simulink model "PV_MEV_FFT_HGQ_BLS"  (R2025a)
settings: Solver=VariableStepAuto  StartTime=0.0  StopTime=0.15  RelTol=1e-3
InitFcn:
  | init_paras
model workspace (MAT data in the model file):
  atk_params = [0 1 0.08 999 0 50 0 0]
values from neighbouring files (symbols this model uses):
  C_PFC = 2600e-6    (= 0.0026)    [init_paras.m]
  ENABLE_HIL = 0    [init_paras.m]
  estimation_src = 1    [init_paras.m]
  Fnom = 50    [init_paras.m]
  Fr_I = Fnom*2    (= 100)    [init_paras.m]
  Ki_V = 80    [init_paras.m]
  Kp_I = 0.06    [init_paras.m]
  Kp_V = 0.25    [init_paras.m]
  Kr_I = 2.5    [init_paras.m]
  L_PFC = 600e-6    (= 0.0006)    [init_paras.m]
  Limit_V = 100    [init_paras.m]
  mm_10cycle_points = mm_points_per_cycle * 10    (= 800)    [init_paras.m]
  mm_fund_freq = 50    [init_paras.m]
  mm_points_per_cycle = 80    [init_paras.m]
  RL_PFC = 20e-3    (= 0.02)    [init_paras.m]
  Ro = 22.22    [init_paras.m]
  Ts_Control = 1/Fc    (= 1e-05)    [init_paras.m]
  Ts_Power = 50e-9    (= 5e-08)    [init_paras.m]
  use_d_predict = 1    [init_paras.m]
  use_harmonic = 1    [init_paras.m]
  use_p_predict = 0    [init_paras.m]
  Vnom_ac = 240    [init_paras.m]
undefined symbols (not defined in the file or in its folder): D1, Delta, DiscIntNeverNeededParam
libraries: spsSeriesRLCBranchLib x17, spsMeanLib x16, spsCurrentMeasurementLib x9, spsFourierLib x8, spsTHDLib x8, spsVoltageMeasurementLib x8, spsDiodeLib x7, MyLibrary x6, instrumentlib x6, pycoexlib x6, simulink x6, spsPWMGeneratorDCDCLib x4
(part 6 of 6)

== matlab function PV_MEV_FFT_HGQ_BLS/EV System2/PFC Control/D_predict ==
  data: i_L input; D output; i_ref input; V_in input; Ts input; L_in input; V_o input; theta_pll input; amp_est input; phase_est input; use_harmonic input
function D  = fcn(i_L, i_ref, V_in, Ts, L_in, V_o, theta_pll, amp_est, phase_est, use_harmonic)

    persistent theta_prev;
    if isempty(theta_prev)
        theta_prev = theta_pll;
    end

    % hyper parameters
    track_gain = 0.35;
    damp_gain = 0.015;

    % Optional
    lead_steps = 1.0;


    % Initialisation 
    L = max(L_in, 1e-9);
    Ts_eff = max(Ts, 1e-9);
    Vo = max(abs(V_o), 1.0);
    ui_L = abs(i_L);

    if V_in > 0
        line_sign = 1.0;
    else
        line_sign = -1.0;
    end

    i_ref_signed = line_sign * abs(i_ref);

    plant_gain = line_sign * L / (Vo * Ts_eff);
    D_ff = 1.0 - abs(V_in) / Vo;

    if use_harmonic

        dtheta = atan2(sin(theta_pll - theta_prev), cos(theta_pll - theta_prev));
        theta_prev = theta_pll;

        omega_inst = dtheta / Ts_eff;

        theta_ctrl = theta_pll + omega_inst * Ts_eff * lead_steps;

        A3 = abs(amp_est(2));
        A5 = abs(amp_est(3));
        A7 = abs(amp_est(4));

        phi3 = phase_est(1);
        phi5 = phase_est(2);
        phi7 = phase_est(3);

        phase_sign = 1.0;

        ih3 = A3 * sin(3.0 * theta_ctrl + phase_sign * phi3);
        ih5 = A5 * sin(5.0 * theta_ctrl + phase_sign * phi5);
        ih7 = A7 * sin(7.0 * theta_ctrl + phase_sign * phi7);

        k3 = 1.00;
        k5 = 1.08;
        k7 = 1.00;

        ih_357 = k3 * ih3 + k5 * ih5 + k7 * ih7;

        i_ref_signed = i_ref_signed - ih_357;
    end

    i_err = i_ref_signed - i_L;

    D_corr = plant_gain * track_gain * i_err;
    D_damp = -line_sign * damp_gain * (i_L - i_ref_signed) / ui_L;

    D = D_ff + D_corr + D_damp;
end

== matlab function PV_MEV_FFT_HGQ_BLS/EV System2/PFC Control/Half Cycle Model Prediction/MATLAB Function ==
  data: x input; x_norm output; A output
function [x_norm, A] = CycleNorm(x)
A = max(abs(x));
A = max(A, 1e-6);
x_norm = x / A;

== matlab function PV_MEV_FFT_HGQ_BLS/EV System/PFC Control/D_predict ==
  data: i_L input; D output; i_ref input; V_in input; Ts input; L_in input; V_o input; theta_pll input; amp_est input; phase_est input; use_harmonic input
function D  = fcn(i_L, i_ref, V_in, Ts, L_in, V_o, theta_pll, amp_est, phase_est, use_harmonic)

    persistent theta_prev;
    if isempty(theta_prev)
        theta_prev = theta_pll;
    end

    % hyper parameters
    track_gain = 0.35;
    damp_gain = 0.015;

    % Optional
    lead_steps = 1.0;


    % Initialisation 
    L = max(L_in, 1e-9);
    Ts_eff = max(Ts, 1e-9);
    Vo = max(abs(V_o), 1.0);
    ui_L = max(abs(i_L), 1e-6);

    if V_in > 0
        line_sign = 1.0;
    else
        line_sign = -1.0;
    end

    i_ref_signed = line_sign * abs(i_ref);

    plant_gain = line_sign * L / (Vo * Ts_eff);
    D_ff = 1.0 - abs(V_in) / Vo;

    if use_harmonic

        dtheta = atan2(sin(theta_pll - theta_prev), cos(theta_pll - theta_prev));
        theta_prev = theta_pll;

        omega_inst = dtheta / Ts_eff;

        theta_ctrl = theta_pll + omega_inst * Ts_eff * lead_steps;

        A3 = abs(amp_est(2));
        A5 = abs(amp_est(3));
        A7 = abs(amp_est(4));

        phi3 = phase_est(1);
        phi5 = phase_est(2);
        phi7 = phase_est(3);

        phase_sign = 1.0;

        ih3 = A3 * sin(3.0 * theta_ctrl + phase_sign * phi3);
        ih5 = A5 * sin(5.0 * theta_ctrl + phase_sign * phi5);
        ih7 = A7 * sin(7.0 * theta_ctrl + phase_sign * phi7);

        k3 = 1.00;
        k5 = 1.08;
        k7 = 1.00;

        ih_357 = k3 * ih3 + k5 * ih5 + k7 * ih7;

        i_ref_signed = i_ref_signed - ih_357;
    end

    i_err = i_ref_signed - i_L;

    D_corr = plant_gain * track_gain * i_err;
    D_damp = -line_sign * damp_gain * (i_L - i_ref_signed) / ui_L;

    D = D_ff + D_corr + D_damp;
end

== matlab function PV_MEV_FFT_HGQ_BLS/EV System/PFC Control/fft estimation 1 cycle2/FFT_estimation_1 ==
  data: u input; amp output; phase output; fs input; f0 input
function [amp, phase] = FFT_estimation_1(u, fs, f0)
%#codegen

x = double(u(:));
N = length(x);

h = zeros(4, 1);
h(1) = 1;
h(2) = 3;
h(3) = 5;
h(4) = 7;

X = fft(x);

amp = zeros(4, 1);
phase_abs_sin = zeros(4, 1);
phase = zeros(3, 1);

tol = 1e-12;

for i = 1:4
    harmonicOrder = h(i);

    bin = round(harmonicOrder * f0 * double(N) / fs);

    if bin <= 0 || bin > floor(double(N) / 2)
        amp(i) = 0;
        phase_abs_sin(i) = 0;
    else
        idx = int32(bin + 1);
        C = X(idx);

        if mod(N, 2) == 0 && bin == N / 2
            amp(i) = abs(C) / double(N);
        else
            amp(i) = 2 * abs(C) / double(N);
        end

        if amp(i) < tol
            phase_abs_sin(i) = 0;
        else
            ph_raw = angle(C);

            ph_sin = ph_raw + pi/2;

            phase_abs_sin(i) = atan2(sin(ph_sin), cos(ph_sin));
        end
    end
end

if amp(1) < tol
    phase(1) = 0;
    phase(2) = 0;
    phase(3) = 0;
else
    phase(1) = atan2( ...
        sin(phase_abs_sin(2) - 3 * phase_abs_sin(1)), ...
        cos(phase_abs_sin(2) - 3 * phase_abs_sin(1)) ...
    );

    phase(2) = atan2( ...
        sin(phase_abs_sin(3) - 5 * phase_abs_sin(1)), ...
        cos(phase_abs_sin(3) - 5 * phase_abs_sin(1)) ...
    );

    phase(3) = atan2( ...
        sin(phase_abs_sin(4) - 7 * phase_abs_sin(1)), ...
        cos(phase_abs_sin(4) - 7 * phase_abs_sin(1)) ...
    );
end

end

== matlab function PV_MEV_FFT_HGQ_BLS/EV System/PFC Control/fft estimation 10 cycle2/FFT_estimation ==
  data: u input; amp output; phase output; fs input; f0 input
function [amp, phase] = FFT_estimation(u, fs, f0)
%#codegen

x = double(u(:));
N = length(x);

h = zeros(4, 1);
h(1) = 1;
h(2) = 3;
h(3) = 5;
h(4) = 7;

X = fft(x);

amp = zeros(4, 1);
phase_abs_sin = zeros(4, 1);
phase = zeros(3, 1);

tol = 1e-12;

for i = 1:4
    harmonicOrder = h(i);

    bin = round(harmonicOrder * f0 * double(N) / fs);

    if bin <= 0 || bin > floor(double(N) / 2)
        amp(i) = 0;
        phase_abs_sin(i) = 0;
    else
        idx = int32(bin + 1);
        C = X(idx);

        if mod(N, 2) == 0 && bin == N / 2
            amp(i) = abs(C) / double(N);
        else
            amp(i) = 2 * abs(C) / double(N);
        end

        if amp(i) < tol
            phase_abs_sin(i) = 0;
        else
            ph_raw = angle(C);

            ph_sin = ph_raw + pi/2;

            phase_abs_sin(i) = atan2(sin(ph_sin), cos(ph_sin));
        end
    end
end

if amp(1) < tol
    phase(1) = 0;
    phase(2) = 0;
    phase(3) = 0;
else
    phase(1) = atan2( ...
        sin(phase_abs_sin(2) - 3 * phase_abs_sin(1)), ...
        cos(phase_abs_sin(2) - 3 * phase_abs_sin(1)) ...
    );

    phase(2) = atan2( ...
        sin(phase_abs_sin(3) - 5 * phase_abs_sin(1)), ...
        cos(phase_abs_sin(3) - 5 * phase_abs_sin(1)) ...
    );

    phase(3) = atan2( ...
        sin(phase_abs_sin(4) - 7 * phase_abs_sin(1)), ...
        cos(phase_abs_sin(4) - 7 * phase_abs_sin(1)) ...
    );
end

end

== matlab function PV_MEV_FFT_HGQ_BLS/EV System/PFC Control/One  Cycle Model Prediction/MATLAB Function ==
  data: x input; x_norm output; A output
function [x_norm, A] = CycleNorm(x)
A = max(abs(x));
A = max(A, 1e-6);
x_norm = x / A;

== matlab function PV_MEV_FFT_HGQ_BLS/EV System2/PFC Control/Half Cycle Model Prediction/MATLAB Function3 ==
  data: y_rel input; y_post output; A_latest input; alpha input; reset input
function y_post = harmonic_postprocess(y_rel, A_latest, alpha, reset)
%#codegen
% 一体化后处理：
% 1) EMA 平滑（在相对输出域）
% 2) A 恢复（幅值乘 A）
% 3) atan2 恢复相位（由 cos/sin -> phase）
%
% 输入:
%   y_rel    : 模型输出(10x1 或 1x10)
%              [amp_h1_rel, amp_h3_rel, amp_h5_rel, amp_h7_rel, ...
%               cos_h3, sin_h3, cos_h5, sin_h5, cos_h7, sin_h7]
%   A_latest : A 恢复系数（可标量或向量；向量时自动取 max(abs(.))）
%   alpha    : EMA 系数 [0,1]，建议 0.10~0.16
%   reset    : 复位信号（true 时重置 EMA 状态）
%
% 输出:
%   y_post(7x1):
%   [amp_h1_abs, amp_h3_abs, amp_h5_abs, amp_h7_abs, phase_h3, phase_h5, phase_h7]

persistent ema_state initialized
if isempty(initialized)
    ema_state = zeros(10,1,'single');
    initialized = false;
end

% -------- 参数/输入整理 --------
y = zeros(10,1,'single');
for i = 1:10
    y(i) = single(y_rel(i));
end

a = single(abs(A_latest));
if numel(a) > 1
    a = max(a(:));
end
if a < single(1e-6)
    a = single(1e-6);
end

a_ema = single(alpha);
if a_ema < single(0)
    a_ema = single(0);
elseif a_ema > single(1)
    a_ema = single(1);
end

do_reset = (reset ~= 0);

% -------- EMA --------
if ~initialized || do_reset
    ema_state = y;
    initialized = true;
else
    ema_state = a_ema * y + (single(1) - a_ema) * ema_state;
end

% -------- A 恢复（幅值）--------
amp = ema_state(1:4) * a;

% -------- 相位恢复（cos/sin -> atan2）--------
% 先单位化，避免 cos/sin 长度漂移导致相位抖动
c3 = ema_state(5); s3 = ema_state(6);
n3 = sqrt(c3*c3 + s3*s3); if n3 < single(1e-6), n3 = single(1e-6); end
c3 = c3 / n3; s3 = s3 / n3;

c5 = ema_state(7); s5 = ema_state(8);
n5 = sqrt(c5*c5 + s5*s5); if n5 < single(1e-6), n5 = single(1e-6); end
c5 = c5 / n5; s5 = s5 / n5;

c7 = ema_state(9); s7 = ema_state(10);
n7 = sqrt(c7*c7 + s7*s7); if n7 < single(1e-6), n7 = single(1e-6); end
c7 = c7 / n7; s7 = s7 / n7;

ph3 = atan2(s3, c3);
ph5 = atan2(s5, c5);
ph7 = atan2(s7, c7);

% -------- 最终输出（仅最终量）--------
y_post = zeros(7,1,'single');
y_post(1:4) = amp;
y_post(5) = ph3;
y_post(6) = ph5;
y_post(7) = ph7;

end

== matlab function PV_MEV_FFT_HGQ_BLS/EV System2/PFC Control/MCP Function Half bridge1 ==
  data: i_L input; y output; i_ref input; V_in input; Ts input; L_in input; V_o input
function y = fcn(i_L, i_ref, V_in, Ts, L_in, V_o)

    L=2*pi*50*L_in;
    % --- Candidate 1: Switch ON ---
    g_on  = i_L + abs(V_in)*Ts/L;
    e_on  = abs(g_on - i_ref);

    % --- Candidate 2: Switch OFF ---
    g_off = i_L + (abs(V_in)-V_o)*Ts/L;
    e_off = abs(g_off - i_ref);

    % --- MPC Decision: pick action with lower predicted error ---
    if e_on <= e_off
        y = true;
    else
        y = false;
    end

== matlab function PV_MEV_FFT_HGQ_BLS/EV System2/PFC Control/One  Cycle Model Prediction/MATLAB Function ==
  data: x input; x_norm output; A output
function [x_norm, A] = CycleNorm(x)
A = max(abs(x));
A = max(A, 1e-6);
x_norm = x / A;

== matlab function PV_MEV_FFT_HGQ_BLS/EV System2/PFC Control/One  Cycle Model Prediction/MATLAB Function3 ==
  data: y_rel input; y_post output; A_latest input; alpha input; reset input
function y_post = harmonic_postprocess(y_rel, A_latest, alpha, reset)
%#codegen
% 一体化后处理：
% 1) EMA 平滑（在相对输出域）
% 2) A 恢复（幅值乘 A）
% 3) atan2 恢复相位（由 cos/sin -> phase）
%
% 输入:
%   y_rel    : 模型输出(10x1 或 1x10)
%              [amp_h1_rel, amp_h3_rel, amp_h5_rel, amp_h7_rel, ...
%               cos_h3, sin_h3, cos_h5, sin_h5, cos_h7, sin_h7]
%   A_latest : A 恢复系数（可标量或向量；向量时自动取 max(abs(.))）
%   alpha    : EMA 系数 [0,1]，建议 0.10~0.16
%   reset    : 复位信号（true 时重置 EMA 状态）
%
% 输出:
%   y_post(7x1):
%   [amp_h1_abs, amp_h3_abs, amp_h5_abs, amp_h7_abs, phase_h3, phase_h5, phase_h7]

persistent ema_state initialized
if isempty(initialized)
    ema_state = zeros(10,1,'single');
    initialized = false;
end

% -------- 参数/输入整理 --------
y = zeros(10,1,'single');
for i = 1:10
    y(i) = single(y_rel(i));
end

a = single(abs(A_latest));
if numel(a) > 1
    a = max(a(:));
end
if a < single(1e-6)
    a = single(1e-6);
end

a_ema = single(alpha);
if a_ema < single(0)
    a_ema = single(0);
elseif a_ema > single(1)
    a_ema = single(1);
end

do_reset = (reset ~= 0);

% -------- EMA --------
if ~initialized || do_reset
    ema_state = y;
    initialized = true;
else
    ema_state = a_ema * y + (single(1) - a_ema) * ema_state;
end

% -------- A 恢复（幅值）--------
amp = ema_state(1:4) * a;

% -------- 相位恢复（cos/sin -> atan2）--------
% 先单位化，避免 cos/sin 长度漂移导致相位抖动
c3 = ema_state(5); s3 = ema_state(6);
n3 = sqrt(c3*c3 + s3*s3); if n3 < single(1e-6), n3 = single(1e-6); end
c3 = c3 / n3; s3 = s3 / n3;

c5 = ema_state(7); s5 = ema_state(8);
n5 = sqrt(c5*c5 + s5*s5); if n5 < single(1e-6), n5 = single(1e-6); end
c5 = c5 / n5; s5 = s5 / n5;

c7 = ema_state(9); s7 = ema_state(10);
n7 = sqrt(c7*c7 + s7*s7); if n7 < single(1e-6), n7 = single(1e-6); end
c7 = c7 / n7; s7 = s7 / n7;

ph3 = atan2(s3, c3);
ph5 = atan2(s5, c5);
ph7 = atan2(s7, c7);

% -------- 最终输出（仅最终量）--------
y_post = zeros(7,1,'single');
y_post(1:4) = amp;
y_post(5) = ph3;
y_post(6) = ph5;
y_post(7) = ph7;

end

== matlab function PV_MEV_FFT_HGQ_BLS/EV System2/PFC Control/RLS_estimation ==
  data: i_L input; amp_est output; theta_pll input; Ts input; reset input; phase_est output; i_h_est output; thdi_est output
function [amp_est, phase_est, i_h_est, thdi_est] = RLS_estimation(i_L, theta_pll, Ts, reset)
%#codegen

nParam = 9;

amp_est = zeros(4, 1);
phase_est = zeros(3, 1);
i_h_est = 0.0;
thdi_est = 0.0;

Ts_eff = max(Ts, 1e-9);

persistent w;
persistent wf;
persistent P;
persistent Ipk_filt;
persistent phase_prev;

if isempty(w) || reset ~= 0
    w = zeros(nParam, 1);
    wf = zeros(nParam, 1);
    P = zeros(nParam, nParam);

    P0 = 250.0;

    for r = 1:nParam
        for c = 1:nParam
            if r == c
                P(r, c) = P0;
            else
                P(r, c) = 0.0;
            end
        end
    end

    Ipk_filt = max(abs(i_L), 1.0);
    phase_prev = zeros(3, 1);
end

Ipk_guard = max(Ipk_filt, 1.0);

tau_est = 0.018;
lambda = exp(-Ts_eff / tau_est);

if lambda < 0.980
    lambda = 0.980;
elseif lambda > 0.99998
    lambda = 0.99998;
end

theta = atan2(sin(theta_pll), cos(theta_pll));

s1 = sin(theta);
c1 = cos(theta);

s3 = sin(3.0 * theta);
c3 = cos(3.0 * theta);

s5 = sin(5.0 * theta);
c5 = cos(5.0 * theta);

s7 = sin(7.0 * theta);
c7 = cos(7.0 * theta);

x = zeros(nParam, 1);

x(1) = 1.0;
x(2) = s1;
x(3) = c1;
x(4) = s3;
x(5) = c3;
x(6) = s5;
x(7) = c5;
x(8) = s7;
x(9) = c7;

y_hat = 0.0;

for k = 1:nParam
    y_hat = y_hat + x(k) * w(k);
end

e = i_L - y_hat;

e_lim = 0.25 * Ipk_guard;

if e_lim < 0.5
    e_lim = 0.5;
end

if e > e_lim
    e = e_lim;
elseif e < -e_lim
    e = -e_lim;
end

Px = zeros(nParam, 1);

for r = 1:nParam
    acc = 0.0;

    for c = 1:nParam
        acc = acc + P(r, c) * x(c);
    end

    Px(r) = acc;
end

xTPx = 0.0;

for k = 1:nParam
    xTPx = xTPx + x(k) * Px(k);
end

den = lambda + xTPx;

if den < 1e-9
    den = 1e-9;
end

K = zeros(nParam, 1);

for k = 1:nParam
    K(k) = Px(k) / den;
end

for k = 1:nParam
    w(k) = w(k) + K(k) * e;
end

for r = 1:nParam
    for c = 1:nParam
        P(r, c) = (P(r, c) - K(r) * Px(c)) / lambda;
    end
end

for r = 1:nParam
    for c = 1:nParam
        if c > r
            p_avg = 0.5 * (P(r, c) + P(c, r));
            P(r, c) = p_avg;
            P(c, r) = p_avg;
        end
    end
end

Pmax = 1e5;
Pmin = 1e-7;

for k = 1:nParam
    if P(k, k) > Pmax
        P(k, k) = Pmax;
    elseif P(k, k) < Pmin
        P(k, k) = Pmin;
    end
end

tau_out = 0.004;
alpha_w = 1.0 - exp(-Ts_eff / tau_out);

if alpha_w < 0.001
    alpha_w = 0.001;
elseif alpha_w > 0.10
    alpha_w = 0.10;
end

for k = 1:nParam
    wf(k) = (1.0 - alpha_w) * wf(k) + alpha_w * w(k);
end

a1 = wf(2);
b1 = wf(3);

a3 = wf(4);
b3 = wf(5);

a5 = wf(6);
b5 = wf(7);

a7 = wf(8);
b7 = wf(9);

A1 = sqrt(a1 * a1 + b1 * b1);
A3 = sqrt(a3 * a3 + b3 * b3);
A5 = sqrt(a5 * a5 + b5 * b5);
A7 = sqrt(a7 * a7 + b7 * b7);

Ipk_now = max(abs(i_L), A1);

if Ipk_now > Ipk_filt
    Ipk_filt = 0.05 * Ipk_now + 0.95 * Ipk_filt;
else
    Ipk_filt = 0.002 * Ipk_now + 0.998 * Ipk_filt;
end

Ipk = max(Ipk_filt, 1e-6);

A1_lim = 1.50 * Ipk;
A3_lim = 0.20 * Ipk;
A5_lim = 0.20 * Ipk;
A7_lim = 0.20 * Ipk;

if A1 > A1_lim
    A1 = A1_lim;
end

if A3 > A3_lim
    A3 = A3_lim;
end

if A5 > A5_lim
    A5 = A5_lim;
end

if A7 > A7_lim
    A7 = A7_lim;
end

phase_min = 0.0015 * Ipk;

if A3 > phase_min
    phi3 = atan2(b3, a3);
    phase_prev(1) = phi3;
else
    phi3 = phase_prev(1);
end

if A5 > phase_min
    phi5 = atan2(b5, a5);
    phase_prev(2) = phi5;
else
    phi5 = phase_prev(2);
end

if A7 > phase_min
    phi7 = atan2(b7, a7);
    phase_prev(3) = phi7;
else
    phi7 = phase_prev(3);
end

phi3 = atan2(sin(phi3), cos(phi3));
phi5 = atan2(sin(phi5), cos(phi5));
phi7 = atan2(sin(phi7), cos(phi7));

amp_est(1) = A1;
amp_est(2) = A3;
amp_est(3) = A5;
amp_est(4) = A7;

phase_est(1) = phi3;
phase_est(2) = phi5;
phase_est(3) = phi7;

i_h_est = a3 * s3 + b3 * c3 + a5 * s5 + b5 * c5 + a7 * s7 + b7 * c7;

if A1 > 1e-6
    thdi_est = sqrt(A3 * A3 + A5 * A5 + A7 * A7) / A1;
else
    thdi_est = 0.0;
end

end

== matlab function PV_MEV_FFT_HGQ_BLS/EV System2/PFC Control/UMPC Function Full bridge1 ==
  data: i_L input; y output; i_ref input; V_in input; Ts input; L_in input; V_o input; g_on output; g_off output
function [y,g_on,g_off]= fcn(i_L, i_ref, V_in, Ts, L_in, V_o)

    L=L_in;

    if V_in >= 0
        i_ref_signed = i_ref;
    else
        i_ref_signed = -i_ref;
    end;

    % -- Positive half Cycle
    if V_in >0
        % --- Candidate 1: Switch ON ---
        g_on  = i_L + (V_in)*Ts/L;
        e_on  = abs(g_on - i_ref_signed);
        
        % --- Candidate 2: Switch OFF ---
        g_off = i_L + (V_in - V_o)*Ts/L;
        e_off = abs(g_off - i_ref_signed);

     % -- Negative half Cycle
    else
        % --- Candidate 1: Switch ON ---
        g_on  = i_L + (V_in)*Ts/L;
        e_on  = abs(g_on - i_ref_signed);

        % --- Candidate 2: Switch OFF ---
        g_off = i_L + (V_in + V_o)*Ts/L;
        e_off = abs(g_off - i_ref_signed);
    end

    % --- MPC Decision: pick action with lower predicted error ---
    if e_on <= e_off
        y = true;
    else
        y = false;
    end

== matlab function PV_MEV_FFT_HGQ_BLS/EV System2/PFC Control/fft estimation 1 cycle2/FFT_estimation_1 ==
  data: u input; amp output; phase output; fs input; f0 input
function [amp, phase] = FFT_estimation_1(u, fs, f0)
%#codegen

x = double(u(:));
N = length(x);

h = zeros(4, 1);
h(1) = 1;
h(2) = 3;
h(3) = 5;
h(4) = 7;

X = fft(x);

amp = zeros(4, 1);
phase_abs_sin = zeros(4, 1);
phase = zeros(3, 1);

tol = 1e-12;

for i = 1:4
    harmonicOrder = h(i);

    bin = round(harmonicOrder * f0 * double(N) / fs);

    if bin <= 0 || bin > floor(double(N) / 2)
        amp(i) = 0;
        phase_abs_sin(i) = 0;
    else
        idx = int32(bin + 1);
        C = X(idx);

        if mod(N, 2) == 0 && bin == N / 2
            amp(i) = abs(C) / double(N);
        else
            amp(i) = 2 * abs(C) / double(N);
        end

        if amp(i) < tol
            phase_abs_sin(i) = 0;
        else
            ph_raw = angle(C);

            ph_sin = ph_raw + pi/2;

            phase_abs_sin(i) = atan2(sin(ph_sin), cos(ph_sin));
        end
    end
end

if amp(1) < tol
    phase(1) = 0;
    phase(2) = 0;
    phase(3) = 0;
else
    phase(1) = atan2( ...
        sin(phase_abs_sin(2) - 3 * phase_abs_sin(1)), ...
        cos(phase_abs_sin(2) - 3 * phase_abs_sin(1)) ...
    );

    phase(2) = atan2( ...
        sin(phase_abs_sin(3) - 5 * phase_abs_sin(1)), ...
        cos(phase_abs_sin(3) - 5 * phase_abs_sin(1)) ...
    );

    phase(3) = atan2( ...
        sin(phase_abs_sin(4) - 7 * phase_abs_sin(1)), ...
        cos(phase_abs_sin(4) - 7 * phase_abs_sin(1)) ...
    );
end

end

== matlab function PV_MEV_FFT_HGQ_BLS/EV System2/PFC Control/fft estimation 10 cycle2/FFT_estimation ==
  data: u input; amp output; phase output; fs input; f0 input
function [amp, phase] = FFT_estimation(u, fs, f0)
%#codegen

x = double(u(:));
N = length(x);

h = zeros(4, 1);
h(1) = 1;
h(2) = 3;
h(3) = 5;
h(4) = 7;

X = fft(x);

amp = zeros(4, 1);
phase_abs_sin = zeros(4, 1);
phase = zeros(3, 1);

tol = 1e-12;

for i = 1:4
    harmonicOrder = h(i);

    bin = round(harmonicOrder * f0 * double(N) / fs);

    if bin <= 0 || bin > floor(double(N) / 2)
        amp(i) = 0;
        phase_abs_sin(i) = 0;
    else
        idx = int32(bin + 1);
        C = X(idx);

        if mod(N, 2) == 0 && bin == N / 2
            amp(i) = abs(C) / double(N);
        else
            amp(i) = 2 * abs(C) / double(N);
        end

        if amp(i) < tol
            phase_abs_sin(i) = 0;
        else
            ph_raw = angle(C);

            ph_sin = ph_raw + pi/2;

            phase_abs_sin(i) = atan2(sin(ph_sin), cos(ph_sin));
        end
    end
end

if amp(1) < tol
    phase(1) = 0;
    phase(2) = 0;
    phase(3) = 0;
else
    phase(1) = atan2( ...
        sin(phase_abs_sin(2) - 3 * phase_abs_sin(1)), ...
        cos(phase_abs_sin(2) - 3 * phase_abs_sin(1)) ...
    );

    phase(2) = atan2( ...
        sin(phase_abs_sin(3) - 5 * phase_abs_sin(1)), ...
        cos(phase_abs_sin(3) - 5 * phase_abs_sin(1)) ...
    );

    phase(3) = atan2( ...
        sin(phase_abs_sin(4) - 7 * phase_abs_sin(1)), ...
        cos(phase_abs_sin(4) - 7 * phase_abs_sin(1)) ...
    );
end

end

== matlab function PV_MEV_FFT_HGQ_BLS/EV System/PFC Control/HGQ FFT-DL Hybrid ==
  data: fft_amplitude input single size=[4 1]; amplitude_out output single size=[4 1]; fft_phase input single size=[3 1]; dl_amplitude input single size=[4 1]; dl_phase input single size=[3 1]; alpha input single size=[4 1]; minimum_ratio input single size=1; phase_out output single size=[3 1]; dl_accepted output boolean size=1
function [amplitude_out, phase_out, dl_accepted] = harmonic_hybrid_fusion_block( ...
    fft_amplitude, fft_phase, dl_amplitude, dl_phase, alpha, minimum_ratio)
%#codegen
% Fuse legacy FFT/DL harmonic estimates in Cartesian coordinates.

amplitude_out = zeros(4, 1, 'single');
phase_out = zeros(3, 1, 'single');
dl_accepted = false;

fft_amp = zeros(4, 1, 'single');
dl_amp = zeros(4, 1, 'single');
weight = zeros(4, 1, 'single');
fft_phi = zeros(3, 1, 'single');
dl_phi = zeros(3, 1, 'single');
for index = 1:4
    fft_amp(index) = single(fft_amplitude(index));
    dl_amp(index) = single(dl_amplitude(index));
    weight(index) = min(max(single(alpha(index)), single(0)), single(1));
end
for index = 1:3
    fft_phi(index) = single(fft_phase(index));
    dl_phi(index) = single(dl_phase(index));
end
ratio = max(single(minimum_ratio), single(0));

valid = true;
for index = 1:4
    valid = valid && isfinite(dl_amp(index)) && dl_amp(index) >= single(0);
end
for index = 1:3
    valid = valid && isfinite(dl_phi(index));
end
valid = valid && dl_amp(1) > single(1e-5);
valid = valid && max(dl_amp(2:4)) <= single(4) * max(dl_amp(1), single(1e-5));

if ~valid
    amplitude_out = fft_amp;
    phase_out = fft_phi;
    return
end
dl_accepted = true;
amplitude_out(1) = (single(1) - weight(1)) * fft_amp(1) + weight(1) * dl_amp(1);
for index = 1:3
    harmonic = index + 1;
    real_part = (single(1) - weight(harmonic)) * fft_amp(harmonic) * cos(fft_phi(index)) ...
        + weight(harmonic) * dl_amp(harmonic) * cos(dl_phi(index));
    imag_part = (single(1) - weight(harmonic)) * fft_amp(harmonic) * sin(fft_phi(index)) ...
        + weight(harmonic) * dl_amp(harmonic) * sin(dl_phi(index));
    amplitude_out(harmonic) = hypot(real_part, imag_part);
    phase_out(index) = atan2(imag_part, real_part);
    if amplitude_out(harmonic) < ratio * max(amplitude_out(1), single(1e-5))
        amplitude_out(harmonic) = single(0);
        phase_out(index) = fft_phi(index);
    end
end
end

== matlab function PV_MEV_FFT_HGQ_BLS/EV System/PFC Control/UMPC Function Full bridge1 ==
  data: i_L input; y output; i_ref input; V_in input; Ts input; L_in input; V_o input; g_on output; g_off output
function [y,g_on,g_off]= fcn(i_L, i_ref, V_in, Ts, L_in, V_o)

    L=L_in;

    if V_in >= 0
        i_ref_signed = i_ref;
    else
        i_ref_signed = -i_ref;
    end;

    % -- Positive half Cycle
    if V_in >0
        % --- Candidate 1: Switch ON ---
        g_on  = i_L + (V_in)*Ts/L;
        e_on  = abs(g_on - i_ref_signed);
        
        % --- Candidate 2: Switch OFF ---
        g_off = i_L + (V_in - V_o)*Ts/L;
        e_off = abs(g_off - i_ref_signed);

     % -- Negative half Cycle
    else
        % --- Candidate 1: Switch ON ---
        g_on  = i_L + (V_in)*Ts/L;
        e_on  = abs(g_on - i_ref_signed);

        % --- Candidate 2: Switch OFF ---
        g_off = i_L + (V_in + V_o)*Ts/L;
        e_off = abs(g_off - i_ref_signed);
    end

    % --- MPC Decision: pick action with lower predicted error ---
    if e_on <= e_off
        y = true;
    else
        y = false;
    end

== matlab function PV_MEV_FFT_HGQ_BLS/EV System/PFC Control/One  Cycle Model Prediction/MATLAB Function3 ==
  data: y_encoded input size=[1 8]; y_post output size=[7 1]; window_peak input size=1; ema_alpha input size=1; reset input size=1
function y_post = harmonic_postprocess8_block(y_encoded, window_peak, ema_alpha, reset)
%#codegen
% Decode [c1,s1,c3,s3,c5,s5,c7,s7] to the legacy MPCC vector:
% [A1,A3,A5,A7,delta3,delta5,delta7].

persistent state initialized
if isempty(initialized)
    state = zeros(8, 1, 'single');
    initialized = false;
end

y = zeros(8, 1, 'single');
for index = 1:8
    y(index) = single(y_encoded(index));
end
alpha = min(max(single(ema_alpha), single(0)), single(1));
if ~initialized || reset ~= 0
    state = y;
    initialized = true;
else
    state = alpha * y + (single(1) - alpha) * state;
end

peak = max(abs(single(window_peak)), single(1e-6));
order_scale = single([1.0; 0.25; 0.20; 0.15]);
amplitude = zeros(4, 1, 'single');
phase = zeros(4, 1, 'single');
for harmonic_index = 1:4
    component = 2 * harmonic_index - 1;
    real_part = state(component);
    imag_part = state(component + 1);
    amplitude(harmonic_index) = peak * order_scale(harmonic_index) * hypot(real_part, imag_part);
    phase(harmonic_index) = atan2(imag_part, real_part);
end

orders = single([3; 5; 7]);
y_post = zeros(7, 1, 'single');
y_post(1:4) = amplitude;
for index = 1:3
    relative = phase(index + 1) - orders(index) * phase(1);
    y_post(index + 4) = atan2(sin(relative), cos(relative));
end
end

== matlab function PV_MEV_FFT_HGQ_BLS/EV System/PFC Control/Half Cycle Model Prediction/MATLAB Function ==
  data: x input; x_norm output; A output
function [x_norm, A] = CycleNorm(x)
A = max(abs(x));
A = max(A, 1e-6);
x_norm = x / A;

== matlab function PV_MEV_FFT_HGQ_BLS/EV System/PFC Control/Half Cycle Model Prediction/MATLAB Function3 ==
  data: y_rel input; y_post output; A_latest input; alpha input; reset input
function y_post = harmonic_postprocess(y_rel, A_latest, alpha, reset)
%#codegen
% 一体化后处理：
% 1) EMA 平滑（在相对输出域）
% 2) A 恢复（幅值乘 A）
% 3) atan2 恢复相位（由 cos/sin -> phase）
%
% 输入:
%   y_rel    : 模型输出(10x1 或 1x10)
%              [amp_h1_rel, amp_h3_rel, amp_h5_rel, amp_h7_rel, ...
%               cos_h3, sin_h3, cos_h5, sin_h5, cos_h7, sin_h7]
%   A_latest : A 恢复系数（可标量或向量；向量时自动取 max(abs(.))）
%   alpha    : EMA 系数 [0,1]，建议 0.10~0.16
%   reset    : 复位信号（true 时重置 EMA 状态）
%
% 输出:
%   y_post(7x1):
%   [amp_h1_abs, amp_h3_abs, amp_h5_abs, amp_h7_abs, phase_h3, phase_h5, phase_h7]

persistent ema_state initialized
if isempty(initialized)
    ema_state = zeros(10,1,'single');
    initialized = false;
end

% -------- 参数/输入整理 --------
y = zeros(10,1,'single');
for i = 1:10
    y(i) = single(y_rel(i));
end

a = single(abs(A_latest));
if numel(a) > 1
    a = max(a(:));
end
if a < single(1e-6)
    a = single(1e-6);
end

a_ema = single(alpha);
if a_ema < single(0)
    a_ema = single(0);
elseif a_ema > single(1)
    a_ema = single(1);
end

do_reset = (reset ~= 0);

% -------- EMA --------
if ~initialized || do_reset
    ema_state = y;
    initialized = true;
else
    ema_state = a_ema * y + (single(1) - a_ema) * ema_state;
end

% -------- A 恢复（幅值）--------
amp = ema_state(1:4) * a;

% -------- 相位恢复（cos/sin -> atan2）--------
% 先单位化，避免 cos/sin 长度漂移导致相位抖动
c3 = ema_state(5); s3 = ema_state(6);
n3 = sqrt(c3*c3 + s3*s3); if n3 < single(1e-6), n3 = single(1e-6); end
c3 = c3 / n3; s3 = s3 / n3;

c5 = ema_state(7); s5 = ema_state(8);
n5 = sqrt(c5*c5 + s5*s5); if n5 < single(1e-6), n5 = single(1e-6); end
c5 = c5 / n5; s5 = s5 / n5;

c7 = ema_state(9); s7 = ema_state(10);
n7 = sqrt(c7*c7 + s7*s7); if n7 < single(1e-6), n7 = single(1e-6); end
c7 = c7 / n7; s7 = s7 / n7;

ph3 = atan2(s3, c3);
ph5 = atan2(s5, c5);
ph7 = atan2(s7, c7);

% -------- 最终输出（仅最终量）--------
y_post = zeros(7,1,'single');
y_post(1:4) = amp;
y_post(5) = ph3;
y_post(6) = ph5;
y_post(7) = ph7;

end

== matlab function PV_MEV_FFT_HGQ_BLS/EV System/PFC Control/MCP Function Half bridge1 ==
  data: i_L input; y output; i_ref input; V_in input; Ts input; L_in input; V_o input
function y = fcn(i_L, i_ref, V_in, Ts, L_in, V_o)

    L=2*pi*50*L_in;
    % --- Candidate 1: Switch ON ---
    g_on  = i_L + abs(V_in)*Ts/L;
    e_on  = abs(g_on - i_ref);

    % --- Candidate 2: Switch OFF ---
    g_off = i_L + (abs(V_in)-V_o)*Ts/L;
    e_off = abs(g_off - i_ref);

    % --- MPC Decision: pick action with lower predicted error ---
    if e_on <= e_off
        y = true;
    else
        y = false;
    end

== matlab function PV_MEV_FFT_HGQ_BLS/EV System/PFC Control/RLS_estimation ==
  data: i_L input; amp_est output; theta_pll input; Ts input; reset input; phase_est output; i_h_est output; thdi_est output
function [amp_est, phase_est, i_h_est, thdi_est] = RLS_estimation(i_L, theta_pll, Ts, reset)
%#codegen

nParam = 9;

amp_est = zeros(4, 1);
phase_est = zeros(3, 1);
i_h_est = 0.0;
thdi_est = 0.0;

Ts_eff = max(Ts, 1e-9);

persistent w;
persistent wf;
persistent P;
persistent Ipk_filt;
persistent phase_prev;

if isempty(w) || reset ~= 0
    w = zeros(nParam, 1);
    wf = zeros(nParam, 1);
    P = zeros(nParam, nParam);

    P0 = 250.0;

    for r = 1:nParam
        for c = 1:nParam
            if r == c
                P(r, c) = P0;
            else
                P(r, c) = 0.0;
            end
        end
    end

    Ipk_filt = max(abs(i_L), 1.0);
    phase_prev = zeros(3, 1);
end

Ipk_guard = max(Ipk_filt, 1.0);

tau_est = 0.018;
lambda = exp(-Ts_eff / tau_est);

if lambda < 0.980
    lambda = 0.980;
elseif lambda > 0.99998
    lambda = 0.99998;
end

theta = atan2(sin(theta_pll), cos(theta_pll));

s1 = sin(theta);
c1 = cos(theta);

s3 = sin(3.0 * theta);
c3 = cos(3.0 * theta);

s5 = sin(5.0 * theta);
c5 = cos(5.0 * theta);

s7 = sin(7.0 * theta);
c7 = cos(7.0 * theta);

x = zeros(nParam, 1);

x(1) = 1.0;
x(2) = s1;
x(3) = c1;
x(4) = s3;
x(5) = c3;
x(6) = s5;
x(7) = c5;
x(8) = s7;
x(9) = c7;

y_hat = 0.0;

for k = 1:nParam
    y_hat = y_hat + x(k) * w(k);
end

e = i_L - y_hat;

e_lim = 0.25 * Ipk_guard;

if e_lim < 0.5
    e_lim = 0.5;
end

if e > e_lim
    e = e_lim;
elseif e < -e_lim
    e = -e_lim;
end

Px = zeros(nParam, 1);

for r = 1:nParam
    acc = 0.0;

    for c = 1:nParam
        acc = acc + P(r, c) * x(c);
    end

    Px(r) = acc;
end

xTPx = 0.0;

for k = 1:nParam
    xTPx = xTPx + x(k) * Px(k);
end

den = lambda + xTPx;

if den < 1e-9
    den = 1e-9;
end

K = zeros(nParam, 1);

for k = 1:nParam
    K(k) = Px(k) / den;
end

for k = 1:nParam
    w(k) = w(k) + K(k) * e;
end

for r = 1:nParam
    for c = 1:nParam
        P(r, c) = (P(r, c) - K(r) * Px(c)) / lambda;
    end
end

for r = 1:nParam
    for c = 1:nParam
        if c > r
            p_avg = 0.5 * (P(r, c) + P(c, r));
            P(r, c) = p_avg;
            P(c, r) = p_avg;
        end
    end
end

Pmax = 1e5;
Pmin = 1e-7;

for k = 1:nParam
    if P(k, k) > Pmax
        P(k, k) = Pmax;
    elseif P(k, k) < Pmin
        P(k, k) = Pmin;
    end
end

tau_out = 0.004;
alpha_w = 1.0 - exp(-Ts_eff / tau_out);

if alpha_w < 0.001
    alpha_w = 0.001;
elseif alpha_w > 0.10
    alpha_w = 0.10;
end

for k = 1:nParam
    wf(k) = (1.0 - alpha_w) * wf(k) + alpha_w * w(k);
end

a1 = wf(2);
b1 = wf(3);

a3 = wf(4);
b3 = wf(5);

a5 = wf(6);
b5 = wf(7);

a7 = wf(8);
b7 = wf(9);

A1 = sqrt(a1 * a1 + b1 * b1);
A3 = sqrt(a3 * a3 + b3 * b3);
A5 = sqrt(a5 * a5 + b5 * b5);
A7 = sqrt(a7 * a7 + b7 * b7);

Ipk_now = max(abs(i_L), A1);

if Ipk_now > Ipk_filt
    Ipk_filt = 0.05 * Ipk_now + 0.95 * Ipk_filt;
else
    Ipk_filt = 0.002 * Ipk_now + 0.998 * Ipk_filt;
end

Ipk = max(Ipk_filt, 1e-6);

A1_lim = 1.50 * Ipk;
A3_lim = 0.20 * Ipk;
A5_lim = 0.20 * Ipk;
A7_lim = 0.20 * Ipk;

if A1 > A1_lim
    A1 = A1_lim;
end

if A3 > A3_lim
    A3 = A3_lim;
end

if A5 > A5_lim
    A5 = A5_lim;
end

if A7 > A7_lim
    A7 = A7_lim;
end

phase_min = 0.0015 * Ipk;

if A3 > phase_min
    phi3 = atan2(b3, a3);
    phase_prev(1) = phi3;
else
    phi3 = phase_prev(1);
end

if A5 > phase_min
    phi5 = atan2(b5, a5);
    phase_prev(2) = phi5;
else
    phi5 = phase_prev(2);
end

if A7 > phase_min
    phi7 = atan2(b7, a7);
    phase_prev(3) = phi7;
else
    phi7 = phase_prev(3);
end

phi3 = atan2(sin(phi3), cos(phi3));
phi5 = atan2(sin(phi5), cos(phi5));
phi7 = atan2(sin(phi7), cos(phi7));

amp_est(1) = A1;
amp_est(2) = A3;
amp_est(3) = A5;
amp_est(4) = A7;

phase_est(1) = phi3;
phase_est(2) = phi5;
phase_est(3) = phi7;

i_h_est = a3 * s3 + b3 * c3 + a5 * s5 + b5 * c5 + a7 * s7 + b7 * c7;

if A1 > 1e-6
    thdi_est = sqrt(A3 * A3 + A5 * A5 + A7 * A7) / A1;
else
    thdi_est = 0.0;
end

end
